simulink model "purePursuit"  (R2022b)
settings: Solver=VariableStepAuto  StartTime=0.0  StopTime=inf  RelTol=1e-3
undefined symbols (not defined in the file or in its folder): Angular, esc, hz, L, ld, Linear, path
libraries: robotlib x4, dspstat3 x1
settings Model: Creator=kisho  LastModifiedBy=kishor
settings DebuggingCC: UnconnectedInputMsg=warning  UnconnectedOutputMsg=warning  UnconnectedLineMsg=warning
settings ModelReferenceCC: EnableRefExpFcnMdlSchedulingChecks=on
settings RTWCC: DLArmComputeVersion=19.05

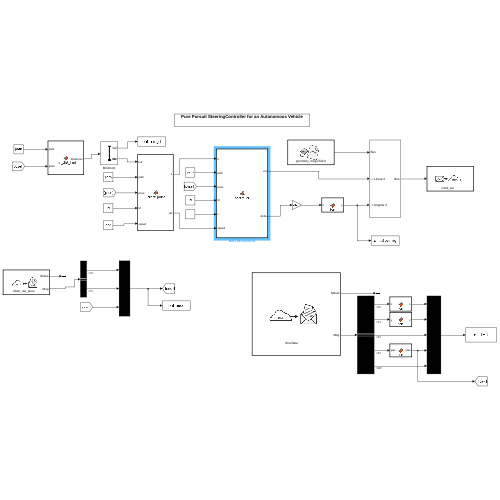
[thumbnail: Simulink's stored preview of the top-level diagram]
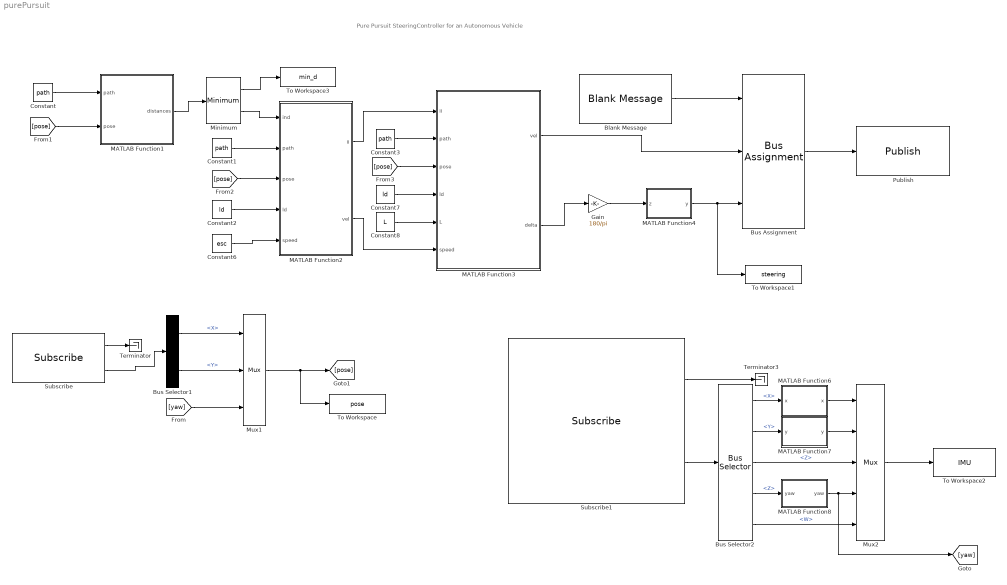
== system purePursuit ==
  note: Pure Pursuit SteeringController for an Autonomous Vehicle
  Blank Message : robotlib/Blank Message  messageClass=Message  entityType=geometry_msgs/Twist  messageType=geometry_msgs/Twist  SampleTime=1/hz  legacyBusStruct=off
      settings: LibrarySourceBlock=roslib/ROS/Blank Message
  Bus Assignment : BusAssignment  AssignedSignals=Linear.X,Angular.Z
  Bus Selector1 : BusSelector  OutputSignals=Pose.Position.X,Pose.Position.Y
  Bus Selector2 : BusSelector  OutputSignals=LinearAcceleration.X,LinearAcceleration.Y,AngularVelocity.Z,Orientation.Z,Orientation.W
  Constant : Constant  Value=path  SampleTime=1/hz
  Constant1 : Constant  Value=path  SampleTime=1/hz
  Constant2 : Constant  Value=ld  SampleTime=1/hz
  Constant3 : Constant  Value=path  SampleTime=1/hz
  Constant6 : Constant  Value=esc  SampleTime=1/hz
  Constant7 : Constant  Value=ld  SampleTime=1/hz
  Constant8 : Constant  Value=L  SampleTime=1/hz
  Gain : Gain  Gain=180/pi
  MATLAB Function1 : MATLAB Function  TreatAsAtomicUnit=on
  MATLAB Function2 : MATLAB Function  TreatAsAtomicUnit=on
  MATLAB Function3 : MATLAB Function  TreatAsAtomicUnit=on
  MATLAB Function4 : MATLAB Function  TreatAsAtomicUnit=on
  MATLAB Function6 : MATLAB Function  TreatAsAtomicUnit=on
  MATLAB Function7 : MATLAB Function  TreatAsAtomicUnit=on
  MATLAB Function8 : MATLAB Function  TreatAsAtomicUnit=on
  Minimum : dspstat3/Minimum  operation=minimum  fcn=Value and Index  indexBase=One  operateOver=Each row  Dimension=1  InputProcessing=Columns as channels (frame based)  reset=None  roiEnable=off  roiType=Rectangles  roiPortion=Entire ROI  roiOutput=Individual statistics for each ROI  roiFlag=off  roundingMode=Floor  overflowMode=off
      settings: LibrarySourceBlock=dsphdlsupportstat/Minimum
  Mux1 : Mux  Inputs=3
  Mux2 : Mux  Inputs=5
  Publish : robotlib/Publish  topicSource=Specify your own  topic=/cmd_vel  messageType=geometry_msgs/Twist  legacyBusStruct=off  messageQueueLength=1
      settings: LibrarySourceBlock=roslib/ROS/Publish
  Subscribe : robotlib/Subscribe  topicSource=Specify your own  topic=/slam_out_pose  messageType=geometry_msgs/PoseStamped  SampleTime=1/hz  legacyBusStruct=off  messageQueueLength=1
      settings: LibrarySourceBlock=roslib/ROS/Subscribe
  Subscribe1 : robotlib/Subscribe  topicSource=Specify your own  topic=/imu/data  messageType=sensor_msgs/Imu  SampleTime=1/hz  legacyBusStruct=off  messageQueueLength=1
      settings: LibrarySourceBlock=roslib/ROS/Subscribe
  Terminator : Terminator
  Terminator3 : Terminator
  To Workspace : ToWorkspace  VariableName=pose  SaveFormat=Structure With Time  SampleTime=-1
  To Workspace1 : ToWorkspace  VariableName=steering  SaveFormat=Structure With Time  SampleTime=1/hz
  To Workspace2 : ToWorkspace  VariableName=IMU  SaveFormat=Structure With Time  SampleTime=-1
  To Workspace3 : ToWorkspace  VariableName=min_d  SaveFormat=Structure With Time  SampleTime=-1
  wires:
  MATLAB Function3/2(delta) -> Gain/1
  Blank Message/1 -> Bus Assignment/1
  Bus Assignment/1 -> Publish/1
  Gain/1 -> MATLAB Function4/1(z)
  MATLAB Function2/1(ii) -> MATLAB Function3/1(ii)
  Constant7/1 -> MATLAB Function3/4(ld)
  Constant1/1 -> MATLAB Function2/2(path)
  Constant3/1 -> MATLAB Function3/2(path)
  [pose] -> MATLAB Function3/3(pose)
  [pose] -> MATLAB Function2/3(pose)
  MATLAB Function1/1(distances) -> Minimum/1
  Minimum/2 -> MATLAB Function2/1(ind)
  Constant2/1 -> MATLAB Function2/4(ld)
  [pose] -> MATLAB Function1/2(pose)
  Constant/1 -> MATLAB Function1/1(path)
  Constant8/1 -> MATLAB Function3/5(L)
  MATLAB Function3/1(vel) -> Bus Assignment/2
  MATLAB Function4/1(y) -> To Workspace1/1, Bus Assignment/3
  Minimum/1 -> To Workspace3/1
  Subscribe/2 -> Bus Selector1/1
  Bus Selector1/2 -> Mux1/2  "<Y>"
  Bus Selector1/1 -> Mux1/1  "<X>"
  Subscribe/1 -> Terminator/1
  Mux1/1 -> [pose], To Workspace/1
  MATLAB Function7/1(y) -> Mux2/2
  Bus Selector2/1 -> MATLAB Function6/1("x ")  "<X>"
  Subscribe1/1 -> Terminator3/1
  Bus Selector2/4 -> MATLAB Function8/1("yaw ")  "<Z>"
  Bus Selector2/2 -> MATLAB Function7/1("y ")  "<Y>"
  MATLAB Function6/1(x) -> Mux2/1
  Subscribe1/2 -> Bus Selector2/1
  Mux2/1 -> To Workspace2/1
  MATLAB Function8/1(yaw) -> [yaw], Mux2/4
  [yaw] -> Mux1/3
  Constant6/1 -> MATLAB Function2/5(speed)
  MATLAB Function2/2(vel) -> MATLAB Function3/6(speed)
  Bus Selector2/3 -> Mux2/3  "<Z>"
  Bus Selector2/5 -> Mux2/5  "<W>"

== matlab function purePursuit/MATLAB Function1 ==
  data: path input; distances output; pose input
function distances  = min_dist_find(path,pose)
 s = length(path);
 dx = zeros(1,s);
 dy = zeros(1,s);
 d  = zeros(1,s);
 for i = 1:s
     dx(i) = path(i,1) - pose(1);
     dy(i) = path(i,2) - pose(2);
 end
 distances = sqrt(dx.^2 + dy.^2);
end

== matlab function purePursuit/MATLAB Function2 ==
  data: ii output; vel output; ind input; path input; pose input; ld input; speed input
function [ii,vel] = Target_point(ind,path,pose,ld,speed)
ii = ind + 1;
vel = speed;
dist = sqrt((path(ii,1)-pose(1))^2 + (path(ii,2)-pose(2))^2);

while (dist<ld)
    ii = ii + 1;
    if ii >= (length(path)-5)
        vel = 0;
    else
        vel = speed;
    end


    dist = sqrt((path(ii,1)-pose(1))^2 + (path(ii,2)-pose(2))^2);
end
end

== matlab function purePursuit/MATLAB Function3 ==
  data: vel output; ii input; delta output; path input; pose input; ld input; L input; speed input
function [vel,delta] = controller(ii,path,pose,ld,L,speed)
%%%%%%%%%%%%%%%%%%%%%%%%%%%%%%%%%%%%%%5

%%%%%%%%%%%%%%%%%%%%%%%%%%%%%%%%%%%%%%%%%%%%

% dx = path(ii,1)- pose(1);
% dy = path(ii,2)- pose(2);
% angle = atan2(dy,dx);
% if(angle < 0)
%     angle = pi + (pi +angle);
% else
% end
% alpha = (angle - pose(3));
% k = 2*sin(alpha)/ld;
% delta = atan(k*L);

%%%%%%%%%%%%%%%%%%%%%%%%%%%%%%%%%%%%%%%%%%%%

dx = path(ii,1)- pose(1);
dy = path(ii,2)- pose(2);
angle = atan2(dy,dx);
if(angle < 0)
    angle = pi + (pi +angle);
else
end
alpha = (angle - pose(3));

if alpha <= -pi
    alpha = angle + (2*pi-pose(3));
elseif alpha >= pi
    alpha = -(2*pi-angle+pose(3));
end

k = 2*sin(alpha)/ld;
delta = atan(k*L);

%%%%%%%%%%%%%%%%%%%%%%%%%%%%%%%%%%%%%%%%%%%%%
vel = speed;

end

== matlab function purePursuit/MATLAB Function4 ==
  data: z input; y output
function y = fcn(z)

if (z > 25)
    z = 25;
elseif (z < -25)
    z = -25;
else
    z =z;
end

y = z;
end

== matlab function purePursuit/MATLAB Function6 ==
  data: x input; x output
function x = fcn(x)
x = x - (0);
end

== matlab function purePursuit/MATLAB Function7 ==
  data: y input; y output
function y = fcn(y)
y = y - (0);
end

== matlab function purePursuit/MATLAB Function8 ==
  data: yaw input; yaw output
function yaw = fcn(yaw)

  yaw = 360-yaw;
  yaw = yaw*pi/180;
end
